simulink model "untitled2"  (R2023b)
settings: Solver=FixedStepAuto  StartTime=0.0  StopTime=15  RelTol=1e-3
values from neighbouring files (symbols this model uses):
  b1 = b(1,:)    [bicyclekinematicmodel.m]
  b2 = b(2,:)    [bicyclekinematicmodel.m]
undefined symbols (not defined in the file or in its folder): a
libraries: fuzblock x1
settings Model: Creator=samee  LastModifiedBy=samee
settings OptimizationCC: EnhancedBackFolding=on  PassReuseOutputArgsAs=Individual arguments  ZeroExternalMemoryAtStartup=off  ZeroInternalMemoryAtStartup=off  MaxStackSize=64  OptimizeBlockOrder=speed  DifferentSizesBufferReuse=on  OptimizationCustomize=off  EfficientTunableParamExpr=on
settings DebuggingCC: ParameterTunabilityLossMsg=error
settings SFSimCC: MATLABDynamicMemAlloc=off
settings RTWCC: Description=Embedded Coder  SystemTargetFile=ert.tlc  HardwareBoard=Robot Operating System 2 (ROS 2)  TLCOptions="-aInlineSetEventsForThisBaseRateFcn=TLC_FALSE -aSuppressMultiTaskScheduler=TLC_FALSE  -aRateBasedStepFcn=0"  TemplateMakefile=ert_default_tmf  Toolchain=Colcon Tools  TargetLang=C++
settings CodeAppCC: ForceParamTrailComments=on  IgnoreCustomStorageClasses=off  OperatorAnnotations=on  SimulinkDataObjDesc=on  SFDataObjDesc=on  InsertBlockDesc=on
settings ERTTargetCC: CodeInterfacePackaging=C++ class  SupportContinuousTime=on  RootIOFormat=Structure reference

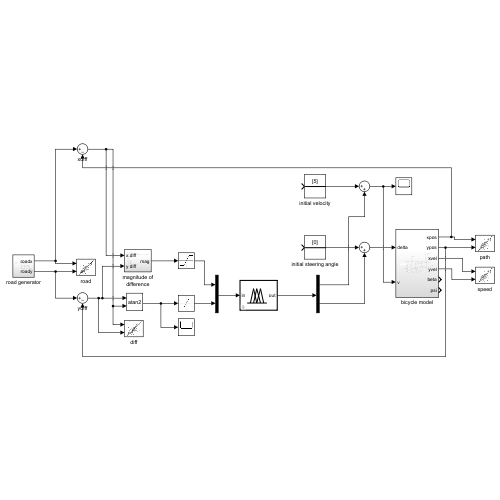
[thumbnail: Simulink's stored preview of the top-level diagram]
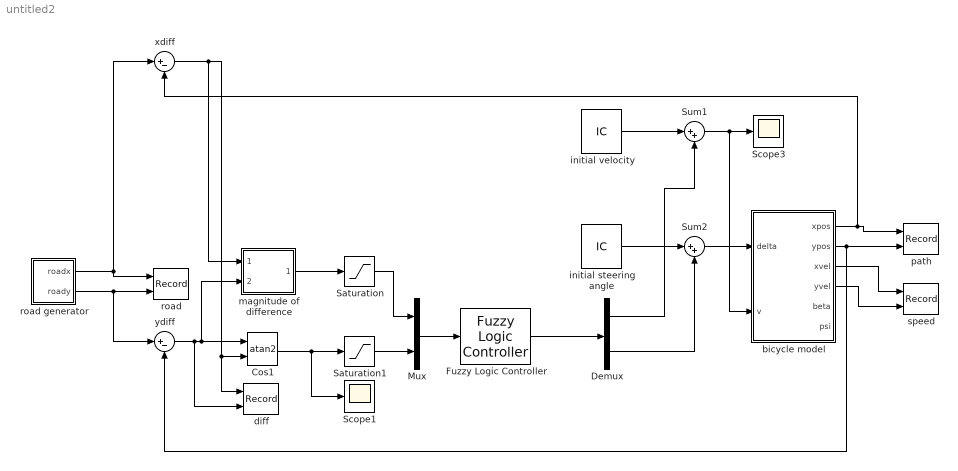
== system untitled2 ==
  Cos1 : Trigonometry  Operator=atan2
  Demux : Demux  Outputs=2
  Fuzzy Logic Controller : fuzblock/Fuzzy Logic  Controller  FIS=fismatrix  OutputSampleNumber=101  DataType=double  FuzzifiedInputs=off  RuleFiringStrengths=off  RuleOutputs=off  AggregatedOutputs=off  SimulateUsing=Interpreted execution  OutOfRangeInputValueMessage=warning  NoRuleFiredMessage=warning  EmptyOutputFuzzySetMessage=warning
  Mux : Mux  Inputs=2
  Saturation : Saturate  UpperLimit=10  LowerLimit=0
  Saturation1 : Saturate  UpperLimit=3.14  LowerLimit=-3.14
  Scope1 : Scope
  Scope3 : Scope
  Sum1 : Sum  Inputs=|++
  Sum2 : Sum  Inputs=|++
  bicycle model : Subsystem
  diff : Record  FileSettingsInternal="{\"entries\":[{\"content\":{\"excelSettings\":{\"content\":{},\"type\":\"Streamout.ExcelSettings\"}},\"type\":\"Streamout.FileSettingStorage\",\"uuid\":\"\"}],\"packageUris\":[\"http:\\/\\/schema.mathworks.com\\/mf0\\/streamout_blocks\\/R2020a\"],\"version\":\"1.0\"}"  Layout=[1 1]  SignalsInternal="{\"entries\":[{\"content\":{\"signals\":[{\"content\":{\"blockPath\":[],\"dimensions\":[1],\"domain\":\"\",\"lineColor\":\"#7e2f8e\",\"plots\":[1],\"port\":1,\"sid\":[\"\"],\"signalID\":2719,\"signalName\":\"xdiff\"},\"type\":\"RecordBlkView.Signal\",\"uuid\":\"\"},{\"content\":{\"blockPath\":[],\"dimensions\":[1],\"domain\":\"\",\"lineColor\":\"#77ac30\",\"plots\":[1],\"port\":2,\"sid\":[\"\"],\"signalID\":2723,\"signalName\":\"ydiff\"},\"type\":\"RecordBlkView.Signal\",\"uuid\":\"\"}]},\"type\":\"RecordBlkView.InputSignals\",\"uuid\":\"\"}],\"packageUris\":[\"http:\\/\\/schema.mathworks.com\\/mf0\\/streamout_blocks\\/R2020a\"],\"version\":\"1.0\"}"  VisualizationBindings="{\"xyplotplugin\":{\"info\":[{\"series\":[{\"bindingParametersList\":[{\"parameter\":\"X-Axis\",\"signalID\":2719,\"signalName\":\"xdiff\"},{\"parameter\":\"Y-Axis\",\"signalID\":2723,\"signalName\":\"ydiff\"}],\"seriesID\":7231}],\"subplotID\":1}]}}"  CompatibilityTag=XY
  initial steering angle : InitialCondition  Value=0
  initial velocity : InitialCondition  Value=5
  magnitude of difference : Subsystem
  path : Record  FileSettingsInternal="{\"entries\":[{\"content\":{\"excelSettings\":{\"content\":{},\"type\":\"Streamout.ExcelSettings\"}},\"type\":\"Streamout.FileSettingStorage\",\"uuid\":\"\"}],\"packageUris\":[\"http:\\/\\/schema.mathworks.com\\/mf0\\/streamout_blocks\\/R2020a\"],\"version\":\"1.0\"}"  Layout=[1 1]  SignalsInternal="{\"entries\":[{\"content\":{\"signals\":[{\"content\":{\"blockPath\":[],\"dimensions\":[1],\"domain\":\"\",\"lineColor\":\"#ff6929\",\"plots\":[1],\"port\":1,\"sid\":[\"\"],\"signalID\":2727,\"signalName\":\"bicycle model:1\"},\"type\":\"RecordBlkView.Signal\",\"uuid\":\"\"},{\"content\":{\"blockPath\":[],\"dimensions\":[1],\"domain\":\"\",\"lineColor\":\"#b746ff\",\"plots\":[1],\"port\":2,\"sid\":[\"\"],\"signalID\":2731,\"signalName\":\"bicycle model:2\"},\"type\":\"RecordBlkView.Signal\",\"uuid\":\"\"}]},\"type\":\"RecordBlkView.InputSignals\",\"uuid\":\"\"}],\"packageUris\":[\"http:\\/\\/schema.mathworks.com\\/mf0\\/streamout_blocks\\/R2020a\"],\"version\":\"1.0\"}"  VisualizationBindings="{\"xyplotplugin\":{\"info\":[{\"series\":[{\"bindingParametersList\":[{\"parameter\":\"X-Axis\",\"signalID\":2727,\"signalName\":\"bicycle model:1\"},{\"parameter\":\"Y-Axis\",\"signalID\":2731,\"signalName\":\"bicycle model:2\"}],\"seriesID\":30809}],\"subplotID\":1}]}}"  CompatibilityTag=XY
  road : Record  FileSettingsInternal="{\"entries\":[{\"content\":{\"excelSettings\":{\"content\":{},\"type\":\"Streamout.ExcelSettings\"}},\"type\":\"Streamout.FileSettingStorage\",\"uuid\":\"\"}],\"packageUris\":[\"http:\\/\\/schema.mathworks.com\\/mf0\\/streamout_blocks\\/R2020a\"],\"version\":\"1.0\"}"  Layout=[1 1]  SignalsInternal="{\"entries\":[{\"content\":{\"signals\":[{\"content\":{\"blockPath\":[],\"dimensions\":[1],\"domain\":\"\",\"lineColor\":\"#139fff\",\"plots\":[1],\"port\":1,\"sid\":[\"\"],\"signalID\":2735,\"signalName\":\"road generator:1\"},\"type\":\"RecordBlkView.Signal\",\"uuid\":\"\"},{\"content\":{\"blockPath\":[],\"dimensions\":[1],\"domain\":\"\",\"lineColor\":\"#ff6929\",\"plots\":[1],\"port\":2,\"sid\":[\"\"],\"signalID\":2739,\"signalName\":\"road generator:2\"},\"type\":\"RecordBlkView.Signal\",\"uuid\":\"\"}]},\"type\":\"RecordBlkView.InputSignals\",\"uuid\":\"\"}],\"packageUris\":[\"http:\\/\\/schema.mathworks.com\\/mf0\\/streamout_blocks\\/R2020a\"],\"version\":\"1.0\"}"  VisualizationBindings="{\"xyplotplugin\":{\"info\":[{\"series\":[{\"bindingParametersList\":[{\"parameter\":\"X-Axis\",\"signalID\":2735,\"signalName\":\"road generator:1\"},{\"parameter\":\"Y-Axis\",\"signalID\":2739,\"signalName\":\"road generator:2\"}],\"seriesID\":43281}],\"subplotID\":1}]}}"  CompatibilityTag=XY
  road generator : Subsystem
  speed : Record  FileSettingsInternal="{\"entries\":[{\"content\":{\"excelSettings\":{\"content\":{},\"type\":\"Streamout.ExcelSettings\"}},\"type\":\"Streamout.FileSettingStorage\",\"uuid\":\"\"}],\"packageUris\":[\"http:\\/\\/schema.mathworks.com\\/mf0\\/streamout_blocks\\/R2020a\"],\"version\":\"1.0\"}"  Layout=[1 1]  SignalsInternal="{\"entries\":[{\"content\":{\"signals\":[{\"content\":{\"blockPath\":[],\"dimensions\":[1],\"domain\":\"\",\"lineColor\":\"#ff6929\",\"plots\":[1],\"port\":1,\"sid\":[\"\"],\"signalID\":2743,\"signalName\":\"bicycle model:3\"},\"type\":\"RecordBlkView.Signal\",\"uuid\":\"\"},{\"content\":{\"blockPath\":[],\"dimensions\":[1],\"domain\":\"\",\"lineColor\":\"#b746ff\",\"plots\":[1],\"port\":2,\"sid\":[\"\"],\"signalID\":2747,\"signalName\":\"bicycle model:4\"},\"type\":\"RecordBlkView.Signal\",\"uuid\":\"\"}]},\"type\":\"RecordBlkView.InputSignals\",\"uuid\":\"\"}],\"packageUris\":[\"http:\\/\\/schema.mathworks.com\\/mf0\\/streamout_blocks\\/R2020a\"],\"version\":\"1.0\"}"  VisualizationBindings="{\"xyplotplugin\":{\"info\":[{\"series\":[{\"bindingParametersList\":[{\"parameter\":\"X-Axis\",\"signalID\":2743,\"signalName\":\"bicycle model:3\"},{\"parameter\":\"Y-Axis\",\"signalID\":2747,\"signalName\":\"bicycle model:4\"}],\"seriesID\":52273}],\"subplotID\":1}]}}"  CompatibilityTag=XY
  xdiff : Sum  Inputs=|+-
  ydiff : Sum  Inputs=|+-
  wires:
  Cos1/1 -> Saturation1/1, Scope1/1
  Demux/1 -> Sum1/2
  road generator/2(roady) -> ydiff/1, road/2
  road generator/1(roadx) -> road/1, xdiff/1
  xdiff/1 -> Cos1/2, diff/1, magnitude of difference/1(x diff)
  bicycle model/1(xpos) -> xdiff/2, path/1
  ydiff/1 -> magnitude of difference/2(y diff), Cos1/1, diff/2
  magnitude of difference/1(mag) -> Saturation/1
  Saturation1/1 -> Mux/2
  Saturation/1 -> Mux/1
  Mux/1 -> Fuzzy Logic Controller/1
  Fuzzy Logic Controller/1 -> Demux/1
  initial velocity/1 -> Sum1/1
  initial steering angle/1 -> Sum2/1
  bicycle model/4(yvel) -> speed/2
  bicycle model/3(xvel) -> speed/1
  Demux/2 -> Sum2/2
  Sum2/1 -> bicycle model/1(delta)
  Sum1/1 -> Scope3/1, bicycle model/2(v)
  bicycle model/2(ypos) -> ydiff/2, path/2

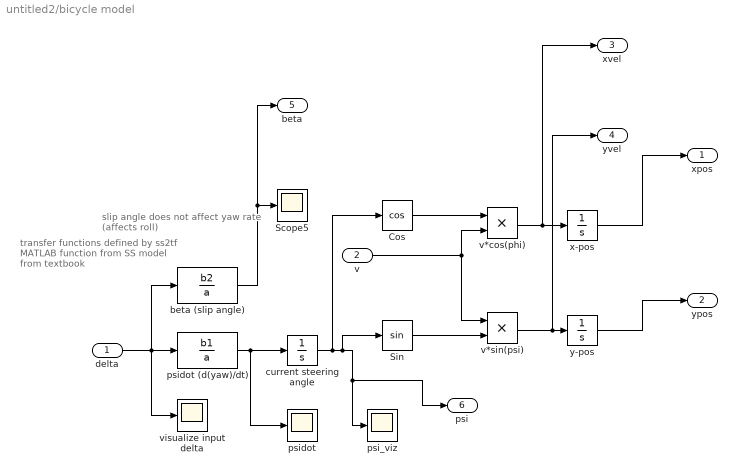
== system untitled2/bicycle model ==
  note: transfer functions defined by ss2tf
      | MATLAB function from SS model
      | from textbook
  note: slip angle does not affect yaw rate
      | (affects roll)
  delta : Inport
  v : Inport  Port=2
  Cos : Trigonometry  Operator=cos
  Scope5 : Scope
  Sin : Trigonometry
  beta (slip angle) : TransferFcn  Numerator=b2  Denominator=a  ContinuousStateAttributes='beta'
  current steering angle : Integrator
  psi_viz : Scope
  psidot : Scope
  psidot (d(yaw)/dt) : TransferFcn  Numerator=b1  Denominator=a  ContinuousStateAttributes='psidot'
  v*cos(phi) : Product
  v*sin(psi) : Product
  visualize input delta : Scope
  x-pos : Integrator
  y-pos : Integrator
  xpos : Outport
  ypos : Outport  Port=2
  xvel : Outport  Port=3
  yvel : Outport  Port=4
  beta : Outport  Port=5
  psi : Outport  Port=6
  wires:
  psidot (d(yaw)/dt)/1 -> current steering angle/1, psidot/1
  v*sin(psi)/1 -> yvel/1, y-pos/1
  current steering angle/1 -> psi/1, psi_viz/1, Sin/1, Cos/1
  delta/1 -> visualize input delta/1, beta (slip angle)/1, psidot (d(yaw)/dt)/1
  Sin/1 -> v*sin(psi)/2
  v/1 -> v*sin(psi)/1, v*cos(phi)/2
  v*cos(phi)/1 -> xvel/1, x-pos/1
  beta (slip angle)/1 -> beta/1, Scope5/1
  Cos/1 -> v*cos(phi)/1
  y-pos/1 -> ypos/1
  x-pos/1 -> xpos/1

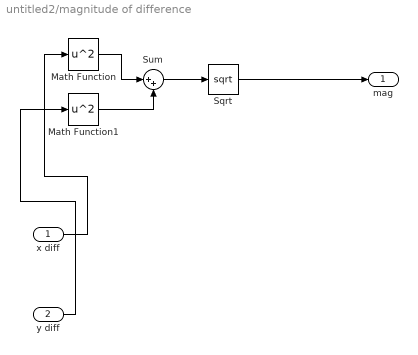
== system untitled2/magnitude of difference ==
  x diff : Inport
  y diff : Inport  Port=2
  Math Function : Math  Operator=square
  Math Function1 : Math  Operator=square
  Sqrt : Sqrt
  Sum : Sum  Inputs=|++
  mag : Outport
  wires:
  Math Function/1 -> Sum/1
  Sum/1 -> Sqrt/1
  Math Function1/1 -> Sum/2
  y diff/1 -> Math Function1/1
  Sqrt/1 -> mag/1
  x diff/1 -> Math Function/1

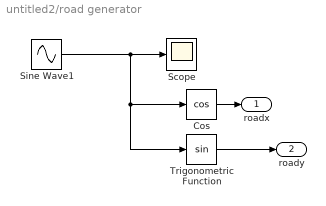
== system untitled2/road generator ==
  Cos : Trigonometry  Operator=cos
  Scope : Scope
  Sine Wave1 : Sin  Frequency=0.25  SampleTime=0
  Trigonometric Function : Trigonometry
  roadx : Outport
  roady : Outport  Port=2
  wires:
  Sine Wave1/1 -> Cos/1, Trigonometric Function/1, Scope/1
  Trigonometric Function/1 -> roady/1
  Cos/1 -> roadx/1
